simulink model "stateflow_transitionUpdate"  (R2015b)
settings: Solver=FixedStepDiscrete  StartTime=0.0  StopTime=10.0  RelTol=1e-3
settings Model: Creator=amyyang  LastModifiedBy=amyyang
settings OptimizationCC: DefaultParameterBehavior=Inlined  OptimizeModelRefInitCode=on  LifeSpan=1
settings RTWCC: SystemTargetFile=ert.tlc  GenCodeOnly=on  TemplateMakefile=ert_default_tmf  Description=Embedded Coder  GenerateReport=on  IncludeHyperlinkInReport=on  LaunchReport=on  GenerateTraceInfo=on  GenerateTraceReport=on  GenerateTraceReportSl=on  GenerateTraceReportSf=on  GenerateTraceReportEml=on
settings CodeAppCC: IgnoreCustomStorageClasses=off
settings ERTTargetCC: GenerateSampleERTMain=on  InlinedParameterPlacement=NonHierarchical  ERTCustomFileTemplate=example_file_process.tlc

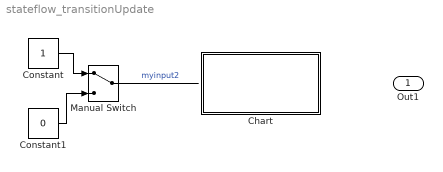
== system stateflow_transitionUpdate ==
  Chart : Stateflow chart  TreatAsAtomicUnit=on
  Constant : Constant
  Constant1 : Constant  Value=0
  Manual Switch : ManualSwitch
  Out1 : Outport
  wires:
  ? -> Out1/1  "out2"
  Manual Switch/1 -> ?  "myinput2"
  Constant/1 -> Manual Switch/1
  Constant1/1 -> Manual Switch/2

== stateflow chart stateflow_transitionUpdate/Chart ==
  settings: updateMethod=DISCRETE  sampleTime=0.1
  state Compare1 [parallel]
    settings: executionOrder=1
    state A
    state B
    (default) -> Compare1.A : {
        |  a = 0;
        | }
    Compare1.B -> Compare1.A : {
        |  a = 0;
        | }
    Compare1.A -> (junction 65) : {
        |  a = addOne(a);
        | }
    (junction 65) -> Compare1.B : [ a >= 8]
  state Compare2 [parallel]
    settings: executionOrder=2
    state A
      du:
      b = addOne(b);
    state B
    (default) -> Compare2.A : {
        |  b = 0;
        | }
    Compare2.B -> Compare2.A : {
        |  b = 0;
        | }
    Compare2.A -> Compare2.B : [ b >=8]
  note: 会出现当b=8时，依然处于状态A
  state y = addOne(x) [function]
    (default) -> (junction 72) : {
        |  y = x + 1;
        | }
  data: x function_input double; y function_output double; a local double; b local double
